simulink model "Blance_ball"  (R2018a)
settings: Solver=ode5  StartTime=0.0  StopTime=3  FixedStep=0.001  RelTol=1e-3
libraries: fuzblock x1
settings Model: Creator=DELL  LastModifiedBy=DELL

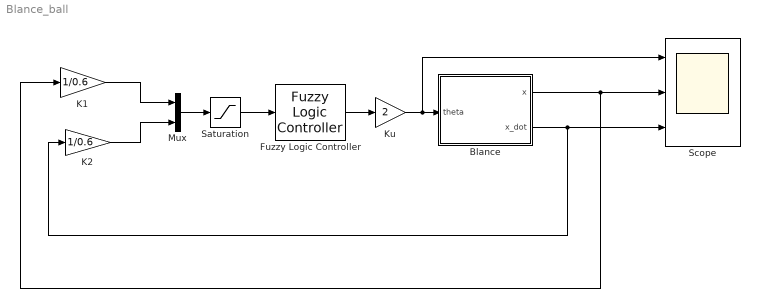
== system Blance_ball ==
  "Blance " : Subsystem  mask{m=0.1, J=0.00005, R=0.02, b=0.005, g=9.81, x_start=-0.3, x_dotstart=-0.3}
      mask prompts: m "mass of ball"; J "momen inertia"; R "radius"; b "coefficient of friction"; g "gravity of acerleration"; x_start "original location"; x_dotstart "initial velocity"
  Fuzzy Logic Controller : fuzblock/Fuzzy Logic  Controller  FIS='balance.fis'  OutputSampleNumber=101  DataType=double  FuzzifiedInputs=off  RuleFiringStrengths=off  RuleOutputs=off  AggregatedOutputs=off  SimulateUsing=Interpreted execution  OutOfRangeInputValueMessage=warning  NoRuleFiredMessage=warning  EmptyOutputFuzzySetMessage=warning
  K1 : Gain  Gain=1/0.6
  K2 : Gain  Gain=1/0.6
  "Ku " : Gain  Gain=2
  Mux : Mux  Inputs=2
  Saturation : Saturate  UpperLimit=1  LowerLimit=-1
  Scope : Scope  NumInputPorts=3
  wires:
  Fuzzy Logic Controller/1 -> "Ku "/1
  "Ku "/1 -> Scope/1, "Blance "/1(theta)
  Saturation/1 -> Fuzzy Logic Controller/1
  Mux/1 -> Saturation/1
  K1/1 -> Mux/1
  K2/1 -> Mux/2
  "Blance "/1(x) -> K1/1, Scope/2
  "Blance "/2(x_dot) -> K2/1, Scope/3

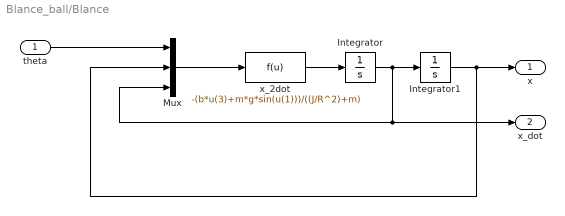
== system Blance_ball/Blance  ==
  theta : Inport
  Integrator : Integrator  InitialCondition=x_dotstart
  Integrator1 : Integrator  InitialCondition=x_start
  Mux : Mux  Inputs=3
  x_2dot : Fcn  Expr=-(b*u(3)+m*g*sin(u(1)))/((J/R^2)+m)
  x : Outport
  x_dot : Outport  Port=2
  wires:
  Integrator/1 -> Mux/3, x_dot/1, Integrator1/1
  x_2dot/1 -> Integrator/1
  theta/1 -> Mux/1
  Mux/1 -> x_2dot/1
  Integrator1/1 -> Mux/2, x/1
